simulink model "Espacio_Estados_Discreto_simulink"  (R2014a)
settings: Solver=VariableStepDiscrete  StartTime=0.0  StopTime=250  RelTol=1e-3
undefined symbols (not defined in the file or in its folder): Ad, Bd, Cd
settings Model: Creator=Jose  LastModifiedBy=Jose

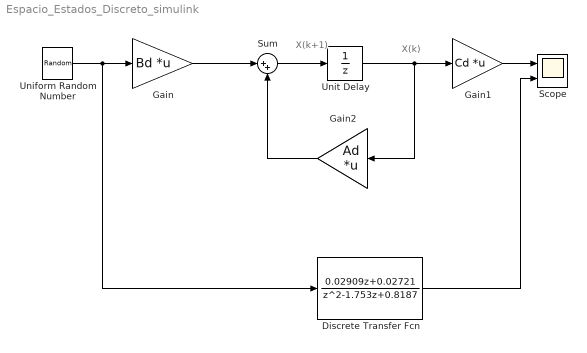
== system Espacio_Estados_Discreto_simulink ==
  note: X(k)
  note: X(k+1)
  Discrete Transfer Fcn : DiscreteTransferFcn  Numerator=[0.02909 0.02721]  Denominator=[1 -1.753 0.8187]  SampleTime=1
  Gain : Gain  Gain=Bd  Multiplication=Matrix(K*u)
  Gain1 : Gain  Gain=Cd  Multiplication=Matrix(K*u)
  Gain2 : Gain  Gain=Ad  Multiplication=Matrix(K*u)
  Scope : Scope  NumInputPorts=2
      settings: YMin=-5~-5  YMax=5~5
  Sum : Sum  Inputs=|++
  Uniform Random Number : UniformRandomNumber  Minimum=0  Maximum=5  SampleTime=50
  Unit Delay : UnitDelay
  wires:
  Gain/1 -> Sum/1
  Sum/1 -> Unit Delay/1
  Unit Delay/1 -> Gain2/1, Gain1/1
  Gain2/1 -> Sum/2
  Uniform Random Number/1 -> Discrete Transfer Fcn/1, Gain/1
  Gain1/1 -> Scope/1
  Discrete Transfer Fcn/1 -> Scope/2
